simulink model "AFCS_1"  (R2016a)
settings: Solver=VariableStepAuto  StartTime=0.0  StopTime=15  RelTol=1e-3
values from neighbouring files (symbols this model uses):
  A = [ ... (first row only)    [AFCS.m]
  B = [ ... (first row only)    [AFCS.m]
  H1 = inv(B'*B)*B'*B1d    [AFCS.m]
  K1 = inv((B'*B))*B'*(A-A1d)    [AFCS.m]
settings Model: Creator=Administrator  LastModifiedBy=Administrator

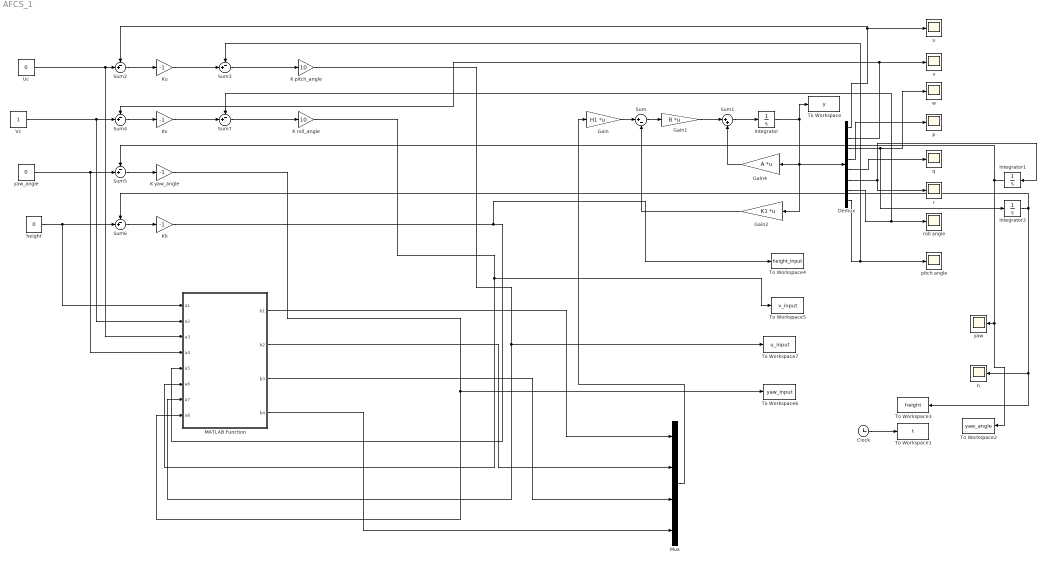
== system AFCS_1 ==
  Clock : Clock
  Demux : Demux  Outputs=8
  Gain : Gain  Gain=H1  Multiplication=Matrix(K*u)
  Gain1 : Gain  Gain=B  Multiplication=Matrix(K*u)
  Gain2 : Gain  Gain=K1  Multiplication=Matrix(K*u)
  Gain4 : Gain  Gain=A  Multiplication=Matrix(K*u)
  Integrator : Integrator
  Integrator1 : Integrator
  Integrator2 : Integrator
  "K pitch_angle " : Gain  Gain=10
  "K roll_angle " : Gain  Gain=10
  K yaw_angle : Gain  Gain=-1
  Kh : Gain  Gain=-1
  Ku : Gain  Gain=-1
  Kv : Gain  Gain=-1
  MATLAB Function : MATLAB Function  TreatAsAtomicUnit=on
  Mux : Mux
  Sum : Sum  Inputs=|+-
  Sum1 : Sum  Inputs=|++
  Sum{2..7} (6 alike) : Sum  Inputs=-+|
  To Workspace : ToWorkspace  VariableName=y  SampleTime=-1
  To Workspace1 : ToWorkspace  VariableName=t  SampleTime=-1
  To Workspace2 : ToWorkspace  VariableName=yaw_angle  SampleTime=-1
  To Workspace3 : ToWorkspace  VariableName=height  SampleTime=-1
  To Workspace4 : ToWorkspace  VariableName=height_input  SampleTime=-1
  To Workspace5 : ToWorkspace  VariableName=v_input  SampleTime=-1
  To Workspace6 : ToWorkspace  VariableName=yaw_input  SampleTime=-1
  To Workspace7 : ToWorkspace  VariableName=u_input  SampleTime=-1
  Uc : Constant  Value=0
  Vc : Constant
  h : Scope
  height : Constant  Value=0
  p : Scope
  pitch angle : Scope
  q : Scope
  r : Scope
  roll angle : Scope
  u : Scope
  v : Scope
  w : Scope
  "yaw " : Scope
  yaw_angle : Constant  Value=0
  wires:
  Mux/1 -> Gain/1
  Gain/1 -> Sum/1
  Sum/1 -> Gain1/1
  Sum1/1 -> Integrator/1
  Integrator/1 -> To Workspace/1, Gain2/1, Gain4/1, Demux/1
  Gain4/1 -> Sum1/2
  Gain2/1 -> Sum/2
  Gain1/1 -> Sum1/1
  Demux/2 -> v/1, Sum4/1
  Demux/3 -> Integrator2/1, w/1
  Demux/4 -> p/1
  Demux/5 -> q/1
  Demux/6 -> r/1, Integrator1/1
  Demux/7 -> Sum7/1, roll angle/1
  Sum2/1 -> Ku/1
  Sum3/1 -> "K pitch_angle "/1
  "K pitch_angle "/1 -> To Workspace7/1, MATLAB Function/7(a7)
  Demux/8 -> pitch angle/1, Sum3/1
  Uc/1 -> MATLAB Function/3(a3), Sum2/2
  Demux/1 -> u/1, Sum2/1
  Clock/1 -> To Workspace1/1
  Ku/1 -> Sum3/2
  Integrator1/1 -> To Workspace2/1, "yaw "/1, Sum5/1
  Vc/1 -> MATLAB Function/2(a2), Sum4/2
  yaw_angle/1 -> MATLAB Function/4(a4), Sum5/2
  height/1 -> MATLAB Function/1(a1), Sum6/2
  Sum4/1 -> Kv/1
  Sum5/1 -> K yaw_angle/1
  Sum6/1 -> Kh/1
  Kv/1 -> Sum7/2
  Sum7/1 -> "K roll_angle "/1
  Kh/1 -> To Workspace4/1, MATLAB Function/5(a5)
  "K roll_angle "/1 -> To Workspace5/1, MATLAB Function/6(a6)
  K yaw_angle/1 -> To Workspace6/1, MATLAB Function/8(a8)
  Integrator2/1 -> Sum6/1, To Workspace3/1, h/1
  MATLAB Function/1(b1) -> Mux/1
  MATLAB Function/2(b2) -> Mux/2
  MATLAB Function/3(b3) -> Mux/3
  MATLAB Function/4(b4) -> Mux/4

== matlab function AFCS_1/MATLAB Function ==
  data: a1 input; b1 output; a2 input; a3 input; a4 input; a5 input; a6 input; a7 input; a8 input; b2 output; b3 output; b4 output
function [b1,b2,b3,b4] = fcn(a1,a2,a3,a4,a5,a6,a7,a8)
%#codegen

if a1~=0
    b1=a5;
    b2=0;
    b3=0;
    b4=0;
    
elseif a2~=0
    b2=a6;
    b1=0;
    b3=0;
    b4=0;
    
elseif a3~=0
    b3=a7;
    b1=0;
    b2=0;
    b4=0;
    
else a4~=0;
    b4=a8;
    b1=0;
    b2=0;
    b3=0;
    
end
